simulink model "cseladd32"  (R2017b)
settings: Solver=ode45  StartTime=0.0  StopTime=1000e-9  FixedStep=0.001  RelTol=1e-3
PostLoadFcn:
  | , if any(exist('dsrtsu_mdlpostloadfcn', 'file') == [2, 3, 6]), try dsrtsu_mdlpostloadfcn('Execute', bdroot); catch fprintf('Error in PostLoadFcn (dsrtsu_mdlpostloadfcn) for model "%s":\n %s\n', bdroot, lasterr); end, end,
libraries: xbsIndex_r4 x17, simulink x2
Description:
  | Standard RTI1005 template.
  | Supported MATLAB version:  R2017b.
settings Model: Tag=RTI1005  DSRTSU_INTERNAL_RTI_VER=540  DSRTSU_INTERNAL_RTI_TYPE=rti1005  RTICANMMDATA=struct('GeneralSetupData',struct('modelroot','C:\Daten\ca72672\Projects\HIL\FPGA_Framework\Playground\DigitalDesign\007_cseladd32','generalsettings',struct('filesettings',struct('destfolder',struct('Name','RTICANMM_FILES','Check',1),'buildfolder',struct('Name','.','Check',1),'AbsDestfolder',struct('Name','C:\Daten\ca72672\Projects\HIL\FPGA_Framework\Playground\DigitalDesign\007_cseladd32\RTICANMM_FILES'),'AbsBuildfolder',struct('Name','C:\Daten\ca72672\Projects\HIL\FPGA_Framework\Playground\DigitalDesign\007_cseladd32'))),'options',struct('addpaths',1,'rmpaths',1,'addtrcexclusion',logical(1),'cannavigator',struct('checkmonitoring',0),'show_usrtrc',0,'use_usrtrc',0),'advanced',struct('options',ones(1,100)),'MPSetup',{{}},'RTI',struct('Type','RTI1005','Ver','7.12','Date','02-May-2019'),'modelname','cseladd32','block','cseladd32'))  DSRTSU_INTERNAL_RTIFPGA=130  Creator=CA72672  LastModifiedBy=CA72672
settings OptimizationCC: BlockReduction=off  OptimizeBlockIOStorage=off  BufferReuse=off  GlobalBufferReuse=off  ExpressionFolding=off  LocalBlockOutputs=off
settings HardwareCC: ProdBitPerPointer=32  ProdBitPerSizeT=32  ProdBitPerPtrDiffT=32  ProdLargestAtomicInteger=Integer  ProdEndianess=BigEndian  ProdWordSize=32  ProdHWDeviceType=Custom Processor->Custom  TargetIntDivRoundTo=Zero  TargetEndianess=BigEndian  TargetHWDeviceType=Custom Processor->Custom
settings SFSimCC: MATLABDynamicMemAlloc=off
settings RTWCC: SystemTargetFile=rti1005.tlc  MakeCommand=make_rti  TemplateMakefile=rti1005.tmf  Description=dSPACE DS1005 Hardware Platform
settings CodeAppCC: StateflowObjectComments=on
settings STFCustomTargetCC: ParMdlRefBuildCompliant=on  MatFileLogging=on  GRTInterface=off  SystemTargetFile=rti1005.tlc
settings GRTTargetCC: TargetLangStandard=C89/C90 (ANSI)  CompOptLevelCompliant=off  ConcurrentExecutionCompliant=off  CombineOutputUpdateFcns=off  CPPClassGenCompliant=off  UseToolchainInfoCompliant=off
settings ConfigComp: CovMetricSettings=dswe

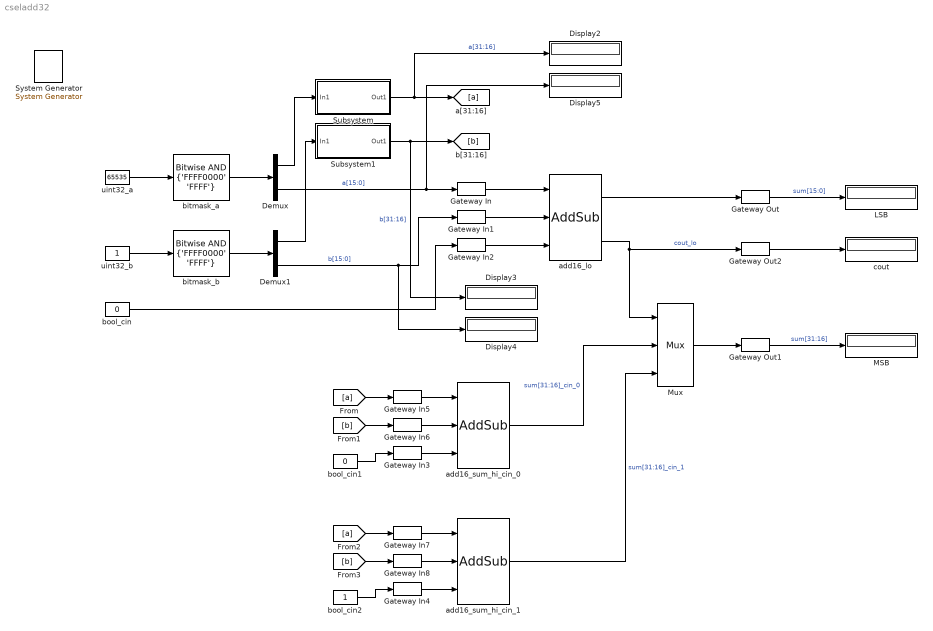
== system cseladd32 ==
  " System Generator" : xbsIndex_r4/ System Generator  Tag=genX  xilinxfamily=kintex7  part=xc7k160t  speed=-1  package=fbg484  synthesis_tool=Vivado  clock_wrapper=Clock Enables  directory=./netlist  proj_type=Vivado  Synth_file=Vivado Synthesis Defaults  Impl_file=Vivado Implementation Defaults  testbench=on  simulink_period=10e-9  sysclk_period=10  dcm_input_clock_period=10  incr_netlist=off  trim_vbits=Everywhere in SubSystem  dbl_ovrd=According to Block Masks  core_generation=According to Block Masks  run_coregen=off  deprecated_control=off  eval_field=0  block_type=sysgen
  Demux : Demux  Outputs=2
  Demux1 : Demux  Outputs=2
  Display{2..5} (4 alike) : Display
  Gateway In{,1,5..8} (6 alike) : xbsIndex_r4/Gateway In  gui_display_data_type=Fixed-point  arith_type=Unsigned  n_bits=16  bin_pt=0  preci_type=Single  exp_width=8  frac_width=24  rows=1  columns=1  quantization="Round  (unbiased: +/- Inf)"  overflow=Wrap  period=10e-9  UseAsADC=off  ADCChannel='1'  interface=None  automatic_assignment=on  address_offset=hex2dec('00')  intf_name=''  intf_description=''  default_value=0  timing_constraint=None  locs_specified=off  LOCs={}  io_standard={}  inherit_from_input=off  hdl_port=on  dbl_ovrd=off  block_type=gatewayin
  Gateway In2 : xbsIndex_r4/Gateway In  gui_display_data_type=Boolean  arith_type=Boolean  n_bits=16  bin_pt=0  preci_type=Single  exp_width=8  frac_width=24  rows=1  columns=1  quantization="Round  (unbiased: +/- Inf)"  overflow=Wrap  period=10e-9  UseAsADC=off  ADCChannel='1'  interface=None  automatic_assignment=on  address_offset=hex2dec('00')  intf_name=''  intf_description=''  default_value=0  timing_constraint=None  locs_specified=off  LOCs={}  io_standard={}  inherit_from_input=off  hdl_port=on  dbl_ovrd=off  block_type=gatewayin
  Gateway In3 : xbsIndex_r4/Gateway In  gui_display_data_type=Boolean  arith_type=Boolean  n_bits=16  bin_pt=0  preci_type=Single  exp_width=8  frac_width=24  rows=1  columns=1  quantization="Round  (unbiased: +/- Inf)"  overflow=Wrap  period=10e-9  UseAsADC=off  ADCChannel='1'  interface=None  automatic_assignment=on  address_offset=hex2dec('00')  intf_name=''  intf_description=''  default_value=0  timing_constraint=None  locs_specified=off  LOCs={}  io_standard={}  inherit_from_input=off  hdl_port=on  dbl_ovrd=off  block_type=gatewayin
  Gateway In4 : xbsIndex_r4/Gateway In  gui_display_data_type=Boolean  arith_type=Boolean  n_bits=16  bin_pt=0  preci_type=Single  exp_width=8  frac_width=24  rows=1  columns=1  quantization="Round  (unbiased: +/- Inf)"  overflow=Wrap  period=10e-9  UseAsADC=off  ADCChannel='1'  interface=None  automatic_assignment=on  address_offset=hex2dec('00')  intf_name=''  intf_description=''  default_value=0  timing_constraint=None  locs_specified=off  LOCs={}  io_standard={}  inherit_from_input=off  hdl_port=on  dbl_ovrd=off  block_type=gatewayin
  Gateway Out : xbsIndex_r4/Gateway Out  inherit_from_input=on  hdl_port=off  rows=1  columns=1  UseAsDAC=off  DACChannel='1'  interface=None  automatic_assignment=on  address_offset=hex2dec('00')  intf_name=''  intf_description=''  timing_constraint=None  locs_specified=off  LOCs={}  io_standard={}  block_type=gatewayout
  Gateway Out1 : xbsIndex_r4/Gateway Out  inherit_from_input=on  hdl_port=off  rows=1  columns=1  UseAsDAC=off  DACChannel='1'  interface=None  automatic_assignment=on  address_offset=hex2dec('00')  intf_name=''  intf_description=''  timing_constraint=None  locs_specified=off  LOCs={}  io_standard={}  block_type=gatewayout
  Gateway Out2 : xbsIndex_r4/Gateway Out  inherit_from_input=on  hdl_port=off  rows=1  columns=1  UseAsDAC=off  DACChannel='1'  interface=None  automatic_assignment=on  address_offset=hex2dec('00')  intf_name=''  intf_description=''  timing_constraint=None  locs_specified=off  LOCs={}  io_standard={}  block_type=gatewayout
  LSB : Display
      settings: Format=hex (Stored Integer)
  MSB : Display
      settings: Format=hex (Stored Integer)
  Mux : xbsIndex_r4/Mux  inputs=2  en=off  latency=1  precision=Full  arith_type=Unsigned  n_bits=16  bin_pt=14  quantization=Truncate  overflow=Wrap  dbl_ovrd=off  block_type=mux
  Subsystem : Subsystem
  Subsystem1 : Subsystem
  add16_lo : xbsIndex_r4/AddSub  mode=Addition  use_carryin=on  use_carryout=on  en=off  latency=16  precision=User Defined  arith_type=Unsigned  n_bits=16  bin_pt=0  quantization=Truncate  overflow=Wrap  use_behavioral_HDL=off  hw_selection=Fabric  pipelined=off  dbl_ovrd=off  block_type=addsub
  add16_sum_hi_cin_0 : xbsIndex_r4/AddSub  mode=Addition  use_carryin=on  use_carryout=off  en=off  latency=16  precision=User Defined  arith_type=Unsigned  n_bits=16  bin_pt=0  quantization="Round  (unbiased: +/- Inf)"  overflow=Wrap  use_behavioral_HDL=off  hw_selection=Fabric  pipelined=off  dbl_ovrd=off  block_type=addsub
  add16_sum_hi_cin_1 : xbsIndex_r4/AddSub  mode=Addition  use_carryin=on  use_carryout=off  en=off  latency=16  precision=User Defined  arith_type=Unsigned  n_bits=16  bin_pt=0  quantization="Round  (unbiased: +/- Inf)"  overflow=Wrap  use_behavioral_HDL=off  hw_selection=Fabric  pipelined=off  dbl_ovrd=off  block_type=addsub
  bitmask_a : simulink/Logic and Bit Operations/Bitwise Operator  logicop=AND  UseBitMask=on  BitMask={'FFFF0000' 'FFFF'}  BitMaskRealWorld=Stored Integer
  bitmask_b : simulink/Logic and Bit Operations/Bitwise Operator  logicop=AND  UseBitMask=on  BitMask={'FFFF0000' 'FFFF'}  BitMaskRealWorld=Stored Integer
  bool_cin : Constant  Value=0  OutDataTypeStr=boolean
  bool_cin1 : Constant  Value=0  OutDataTypeStr=boolean
  bool_cin2 : Constant  OutDataTypeStr=boolean
  cout : Display
  uint32_a : Constant  Value=65535  OutDataTypeStr=uint32
  uint32_b : Constant  OutDataTypeStr=uint32
  wires:
  Demux/2 -> Display5/1, Gateway In/1  "a[15:0]"
  Gateway In/1 -> add16_lo/1
  Gateway In1/1 -> add16_lo/2
  bool_cin/1 -> Gateway In2/1
  Gateway In2/1 -> add16_lo/3
  add16_lo/1 -> Gateway Out/1
  add16_lo/2 -> Gateway Out2/1, Mux/1  "cout_lo"
  uint32_a/1 -> bitmask_a/1
  bitmask_a/1 -> Demux/1
  Demux/1 -> Subsystem/1(In1)
  Demux1/1 -> Subsystem1/1(In1)
  bitmask_b/1 -> Demux1/1
  uint32_b/1 -> bitmask_b/1
  Demux1/2 -> Display4/1, Gateway In1/1  "b[15:0]"
  [a] -> Gateway In5/1
  [b] -> Gateway In6/1
  Gateway In3/1 -> add16_sum_hi_cin_0/3
  bool_cin1/1 -> Gateway In3/1
  bool_cin2/1 -> Gateway In4/1
  Gateway In4/1 -> add16_sum_hi_cin_1/3
  [b] -> Gateway In8/1
  [a] -> Gateway In7/1
  add16_sum_hi_cin_0/1 -> Mux/2  "sum[31:16]_cin_0"
  add16_sum_hi_cin_1/1 -> Mux/3  "sum[31:16]_cin_1"
  Mux/1 -> Gateway Out1/1
  Gateway In5/1 -> add16_sum_hi_cin_0/1
  Gateway In6/1 -> add16_sum_hi_cin_0/2
  Gateway In7/1 -> add16_sum_hi_cin_1/1
  Gateway In8/1 -> add16_sum_hi_cin_1/2
  Gateway Out/1 -> LSB/1  "sum[15:0]"
  Gateway Out1/1 -> MSB/1  "sum[31:16]"
  Subsystem/1(Out1) -> Display2/1, [a]  "a[31:16]"
  Subsystem1/1(Out1) -> Display3/1, [b]  "b[31:16]"
  Gateway Out2/1 -> cout/1

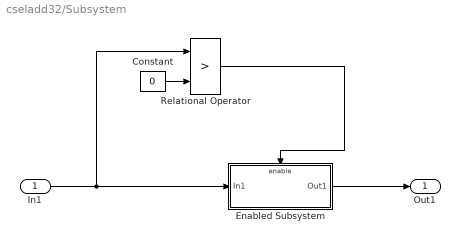
== system cseladd32/Subsystem ==
  In1 : Inport
  Constant : Constant  Value=0
  Enabled Subsystem : Subsystem  TreatAsAtomicUnit=on
  Relational Operator : RelationalOperator  Operator=>  OutDataTypeStr=boolean  RndMeth=Simplest
  Out1 : Outport
  wires:
  Constant/1 -> Relational Operator/2
  Relational Operator/1 -> Enabled Subsystem/Enable
  Enabled Subsystem/1(Out1) -> Out1/1
  In1/1 -> Enabled Subsystem/1(In1), Relational Operator/1

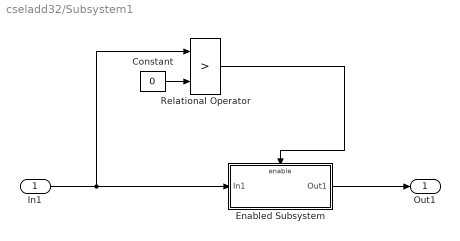
== system cseladd32/Subsystem1 ==
  In1 : Inport
  Constant : Constant  Value=0
  Enabled Subsystem : Subsystem  TreatAsAtomicUnit=on
  Relational Operator : RelationalOperator  Operator=>  OutDataTypeStr=boolean  RndMeth=Simplest
  Out1 : Outport
  wires:
  Enabled Subsystem/1(Out1) -> Out1/1
  In1/1 -> Enabled Subsystem/1(In1), Relational Operator/1
  Relational Operator/1 -> Enabled Subsystem/Enable
  Constant/1 -> Relational Operator/2

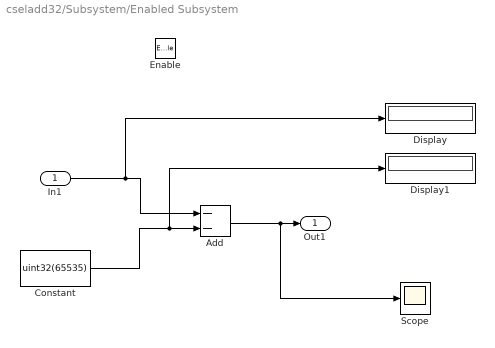
== system cseladd32/Subsystem/Enabled Subsystem ==
  In1 : Inport
  Enable : EnablePort
  Add : Sum  Inputs=--  OutDataTypeStr=uint16
  Constant : Constant  Value=uint32(65535)  OutDataTypeStr=uint32
  Display : Display
  Display1 : Display
  Scope : Scope
  Out1 : Outport
  wires:
  Add/1 -> Scope/1, Out1/1
  In1/1 -> Display/1, Add/1
  Constant/1 -> Display1/1, Add/2

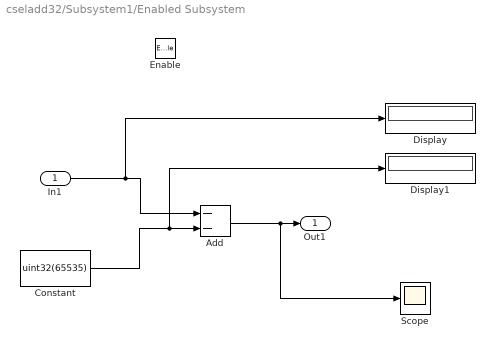
== system cseladd32/Subsystem1/Enabled Subsystem ==
  In1 : Inport
  Enable : EnablePort
  Add : Sum  Inputs=--  OutDataTypeStr=uint16
  Constant : Constant  Value=uint32(65535)  OutDataTypeStr=uint32
  Display : Display
  Display1 : Display
  Scope : Scope
  Out1 : Outport
  wires:
  Add/1 -> Scope/1, Out1/1
  In1/1 -> Display/1, Add/1
  Constant/1 -> Display1/1, Add/2
